simulink model "test"  (R2022b)
settings: Solver=VariableStepAuto  StartTime=0.0  StopTime=30  RelTol=1e-3
values from neighbouring files (symbols this model uses):
  Clq = 1.18    [tavola3.m]
  Clu = 17.24    [tavola3.m]
  Clw = 38.06    [tavola3.m]
  Cqq = 7.51    [tavola3.m]
  Cqu = 106.03    [tavola3.m]
  Cqw = 84.1    [tavola3.m]
  I = [tau_u;0;tau_q]    [tavola2.m]    (also in tavola3.m = 5.98)
  m = 115    [tavola3.m]
settings Model: Creator=morel  LastModifiedBy=morel

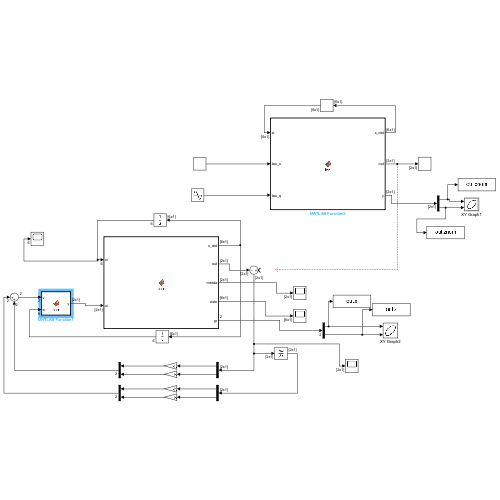
[thumbnail: Simulink's stored preview of the top-level diagram]
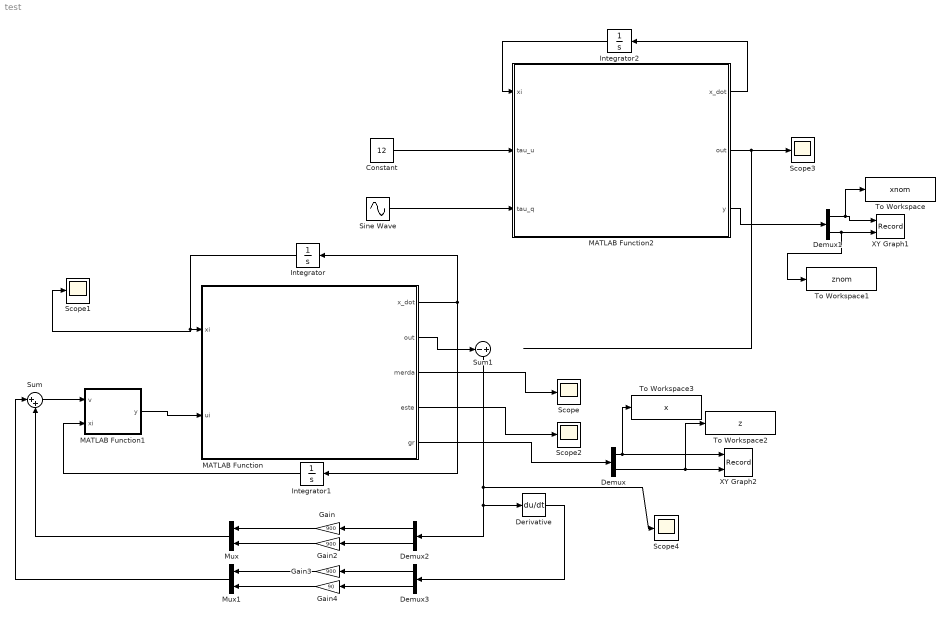
== system test ==
  Constant : Constant  Value=12
  Demux{,1..3} (4 alike) : Demux  Outputs=2
  Derivative : Derivative
  Gain : Gain  Gain=900
  Gain2 : Gain  Gain=900
  Gain3 : Gain  Gain=900
  Gain4 : Gain  Gain=90
  Integrator : Integrator  InitialCondition=[5;-13.5;1.5;0;0;0]
  Integrator1 : Integrator  InitialCondition=zeros(6,1)
  Integrator2 : Integrator  InitialCondition=[0;-10;0;0.1;0;0]
  MATLAB Function : MATLAB Function  TreatAsAtomicUnit=on
  MATLAB Function1 : MATLAB Function  TreatAsAtomicUnit=on
  MATLAB Function2 : MATLAB Function  TreatAsAtomicUnit=on
  Mux : Mux  Inputs=2
  Mux1 : Mux  Inputs=2
  Scope{,1..4} (5 alike) : Scope
  Sine Wave : Sin  Amplitude=0.4  SampleTime=0
  Sum : Sum  Inputs=|++
  Sum1 : Sum  Inputs=-|+
  To Workspace : ToWorkspace  VariableName=xnom  SaveFormat=Timeseries  SampleTime=-1
  To Workspace1 : ToWorkspace  VariableName=znom  SaveFormat=Timeseries  SampleTime=-1
  To Workspace2 : ToWorkspace  VariableName=z  SaveFormat=Timeseries  SampleTime=-1
  To Workspace3 : ToWorkspace  VariableName=x  SaveFormat=Timeseries  SampleTime=-1
  XY Graph1 : Record  FileSettingsInternal="{\"entries\":[{\"content\":{\"excelSettings\":{\"content\":{},\"type\":\"Streamout.ExcelSettings\"}},\"type\":\"Streamout.FileSettingStorage\",\"uuid\":\"0907c80f-1aed-4eb9-80d5-bd6d60abdef0\"}],\"packageUris\":[\"http://schema.mathworks.com/mf0/streamout_blocks/R2020a\"],\"version\":\"1.0\"}"  Layout=[1 1]  SignalsInternal="{\"entries\":[{\"content\":{\"signals\":[{\"content\":{\"blockPath\":[\"test/XY Graph1\"],\"channel\":[],\"dimensions\":[1,1],\"domain\":\"test/XY Graph1\",\"lineColor\":\"#a2142f\",\"plots\":[1],\"port\":1,\"sid\":[\"\"],\"signalID\":2856,\"signalName\":\"Demux1:1\"},\"type\":\"RecordBlkView.Signal\",\"uuid\":\"abc5ec7b-7ef8-4cb9-9d52-9f8f9f7d8ccf\"},{\"content\":{\"blockPath\":[\"test/XY Graph1\"],\"channel\":[],\"dimensions\":[1,1],\"domain\":\"test/XY Graph1\",\"lineColor\":\"#139fff\",\"plots\":[1],\"port\":2,\"sid\":[\"\"],\"signalID\":2860,\"signalName\":\"Demux1:2\"},\"type\":\"RecordBlkView.Signal\",\"uuid\":\"2d3d5a5a-198f-4092-aac2-d6f1e2c588f4\"}]},\"type\":\"RecordBlkView.InputSignals\",\"uuid\":\"2631c857-486c-41e2-bc6a-4e52098b57e7\"}],\"packageUris\":[\"http://schema.mathworks.com/mf0/streamout_blocks/R2020a\"],\"version\":\"1.0\"}"  VisualizationBindings="{\"xyplotplugin\":{\"info\":[{\"series\":[{\"bindingParametersList\":[{\"parameter\":\"X-Axis\",\"signalID\":2856,\"signalName\":\"Demux1:1\"},{\"parameter\":\"Y-Axis\",\"signalID\":2860,\"signalName\":\"Demux1:2\"}],\"seriesID\":41840}],\"subplotID\":1}]}}"  CompatibilityTag=XY
  XY Graph2 : Record  FileSettingsInternal="{\"entries\":[{\"content\":{\"excelSettings\":{\"content\":{},\"type\":\"Streamout.ExcelSettings\"}},\"type\":\"Streamout.FileSettingStorage\",\"uuid\":\"aee596d7-e5fa-465f-bc79-717a28723c84\"}],\"packageUris\":[\"http://schema.mathworks.com/mf0/streamout_blocks/R2020a\"],\"version\":\"1.0\"}"  Layout=[1 1]  SignalsInternal="{\"entries\":[{\"content\":{\"signals\":[{\"content\":{\"blockPath\":[\"test/XY Graph2\"],\"channel\":[],\"dimensions\":[1],\"domain\":\"test/XY Graph2\",\"lineColor\":\"#a2142f\",\"plots\":[1],\"port\":1,\"sid\":[\"\"],\"signalID\":2872,\"signalName\":\"Demux:1\"},\"type\":\"RecordBlkView.Signal\",\"uuid\":\"79364f59-d53f-4e76-9c60-3a2e95498284\"},{\"content\":{\"blockPath\":[\"test/XY Graph2\"],\"channel\":[],\"dimensions\":[1],\"domain\":\"test/XY Graph2\",\"lineColor\":\"#139fff\",\"plots\":[1],\"port\":2,\"sid\":[\"\"],\"signalID\":2876,\"signalName\":\"Demux:2\"},\"type\":\"RecordBlkView.Signal\",\"uuid\":\"0aa172fb-da37-458e-85a1-3a5c731bebe4\"}]},\"type\":\"RecordBlkView.InputSignals\",\"uuid\":\"f3ce4fa0-0bac-449e-9e86-78042f509b2b\"}],\"packageUris\":[\"http://schema.mathworks.com/mf0/streamout_blocks/R2020a\"],\"version\":\"1.0\"}"  VisualizationBindings="{\"xyplotplugin\":{\"info\":[{\"series\":[{\"bindingParametersList\":[{\"parameter\":\"X-Axis\",\"signalID\":2872,\"signalName\":\"Demux:1\"},{\"parameter\":\"Y-Axis\",\"signalID\":2876,\"signalName\":\"Demux:2\"}],\"seriesID\":20199}],\"subplotID\":1}]}}"  CompatibilityTag=XY
  wires:
  MATLAB Function/1(x_dot) -> Integrator1/1, Integrator/1
  Integrator/1 -> Scope1/1, MATLAB Function/1(xi)
  Integrator1/1 -> MATLAB Function1/2(xi)
  MATLAB Function1/1(y) -> MATLAB Function/2(ui)
  Sum/1 -> MATLAB Function1/1(v)
  MATLAB Function/3(merda) -> Scope/1
  MATLAB Function/4(este) -> Scope2/1
  MATLAB Function2/1(x_dot) -> Integrator2/1
  Integrator2/1 -> MATLAB Function2/1(xi)
  Sine Wave/1 -> MATLAB Function2/3(tau_q)
  Constant/1 -> MATLAB Function2/2(tau_u)
  MATLAB Function2/2(out) -> Scope3/1
  MATLAB Function/2(out) -> Sum1/1
  MATLAB Function/5(gr) -> Demux/1
  Demux1/2 -> To Workspace1/1, XY Graph1/2
  MATLAB Function2/3(y) -> Demux1/1
  Sum1/1 -> Demux2/1, Derivative/1, Scope4/1
  Demux2/2 -> Gain2/1
  Demux2/1 -> Gain/1
  Gain2/1 -> Mux/2
  Gain/1 -> Mux/1
  Mux/1 -> Sum/2
  Demux3/2 -> Gain4/1
  Gain4/1 -> Mux1/2
  Gain3/1 -> Mux1/1
  Mux1/1 -> Sum/1
  Demux3/1 -> Gain3/1
  Derivative/1 -> Demux3/1
  Demux/2 -> To Workspace2/1, XY Graph2/2
  Demux/1 -> To Workspace3/1, XY Graph2/1
  Demux1/1 -> To Workspace/1, XY Graph1/1

== matlab function test/MATLAB Function1 ==
  data: v input; xi input; y output; Clu parameter; Cqu parameter; Clq parameter; Cqq parameter; Clw parameter; Cqw parameter; m parameter; I parameter
function y = fcn(v,xi,Clu, Cqu, Clq, Cqq, Clw, Cqw,m,I)

theta = xi(3);
u= xi(4);
w= xi(5);
q= xi(6);
%s = [v(1,1);
  %  wrapTo2Pi(v(1,2))];


 
gamma = [ cos(theta)*(q*u - (w*(Clw + Cqw*abs(w)))/m) - q*(u*cos(theta) + w*sin(theta)) + sin(theta)*(q*w + (u*(Clu + Cqu*abs(u)))/m);
        -(q*(Clq + Cqq*abs(q)))/I];

E = [-sin(theta), 0 ;
      0,         1];

y = -inv(E)*gamma +inv(E)*v;

== matlab function test/MATLAB Function ==
  data: xi input; x_dot output; m parameter; I parameter; Clq parameter; Clw parameter; Clu parameter; Cqw parameter; Cqq parameter; Cqu parameter; ui input; out output; merda output; este output; gr output
function [x_dot,out,merda,este,gr] = fcn(xi,m, I,Clq, Clw, Clu,Cqw, Cqq, Cqu,ui)

x=xi(1);
z=xi(2);
theta = xi(3);
theta=wrapTo2Pi(theta);
u = xi(4);
w = xi(5);
q = xi(6);
tau_u=ui(1);
tau_q=ui(2);

f =[ u*cos(theta) + w*sin(theta);
     w*cos(theta) - u*sin(theta);
                               q;
- q*w - (u*(Clu + Cqu*abs(u)))/m;
  q*u - (w*(Clw + Cqw*abs(w)))/m;
       -(q*(Clq + Cqq*abs(q)))/I];

g1 =[0;
     0;
     0;
     1;
     0;
     0];

g2 =[0;
     0;
     0;
     0;
     0;
     1];



x_dot = f + g1*tau_u + g2*tau_q;






%%%%%%%%%%%%%%%%%%%%%%%%%%%%%%%%%%%%%%%%%%%%%%%%%%%%%%%%%%%5





eta = [z;w];



Q = [0,1;
     0,-(Clw+Cqw*abs(w))/m];




merda = Q*eta;

este = [x;u*cos(theta) + w*sin(theta);theta;q;merda];



%%%%%%%%%%%%%%%%%%%%%%%%%%%%%%%%%%%%%%%%%%%%%%%%%%%%%%%%%%%
out = [z;theta];


gr=[x;z];

== matlab function test/MATLAB Function2 ==
  data: xi input; x_dot output; m parameter; I parameter; Clq parameter; Clw parameter; Clu parameter; Cqw parameter; Cqq parameter; Cqu parameter; tau_u input; out output; tau_q input; y output
function [x_dot,out,y] = fcn(xi,m, I,Clq, Clw, Clu,Cqw, Cqq, Cqu,tau_u,tau_q)

x=xi(1);
z=xi(2);
theta = xi(3);
u = xi(4);
w = xi(5);
q = xi(6);


f =[ u*cos(theta) + w*sin(theta);
     w*cos(theta) - u*sin(theta);
                               q;
- q*w - (u*(Clu + Cqu*abs(u)))/m;
  q*u - (w*(Clw + Cqw*abs(w)))/m;
       -(q*(Clq + Cqq*abs(q)))/I];

g1 =[0;
     0;
     0;
     1;
     0;
     0];

g2 =[0;
     0;
     0;
     0;
     0;
     1];



x_dot = f + g1*tau_u + g2*tau_q;


%%%%%%%%%%%%%%%%%%%%%%%%%%%%%%%%%%%%%%%%%%%%%%%%%%%%%%%%%%%
out = [x;theta];
y = [x;z];
